simulink model "Lab1_parameter_estimation_student"  (R2025a)
settings: Solver=FixedStepAuto  StartTime=0.0  StopTime=20  FixedStep=0.0005  RelTol=1e-3
values from neighbouring files (symbols this model uses):
  motor_B = 3.13337426732843E-06    (= 3.13337426733e-06)    [Lab1_motor_params_student.m]    (also in Params_Chirp.mat = 6.5871616123e-07; Params_Ramp.mat = 8.73861222158e-05; Params_Sine.mat = 8.59415048861e-06; Params_Stair.mat = 3.2047e-05)
  motor_Eff = 0.750882138129295    (= 0.750882138129)    [Lab1_motor_params_student.m]    (also in Params_Chirp.mat = 0.998383269214; Params_Ramp.mat = 0.688800701516; Params_Sine.mat = 0.573625535666; Params_Stair.mat = 0.952868616)
  motor_J = 3.67584411965396E-06    (= 3.67584411965e-06)    [Lab1_motor_params_student.m]    (also in Params_Chirp.mat = 1.17123806047e-05; Params_Ramp.mat = 8.05298799031e-05; Params_Sine.mat = 8.20240322026e-06; Params_Stair.mat = 9.875e-06)
  motor_Ke = 0.0595281219387613    (= 0.0595281219388)    [Lab1_motor_params_student.m]    (also in Params_Chirp.mat = 0.0500817047826; Params_Ramp.mat = 0.0340798970374; Params_Sine.mat = 0.0488089871517; Params_Stair.mat = 0.047996267)
  motor_L = 0.136562826    [Lab1_motor_params_student.m]
  motor_R = 9.393179725    [Lab1_motor_params_student.m]
libraries: simulink x3
settings Model: Creator=tanawatp  LastModifiedBy=User
settings RTWCC: GPUComputeCapability=3.5

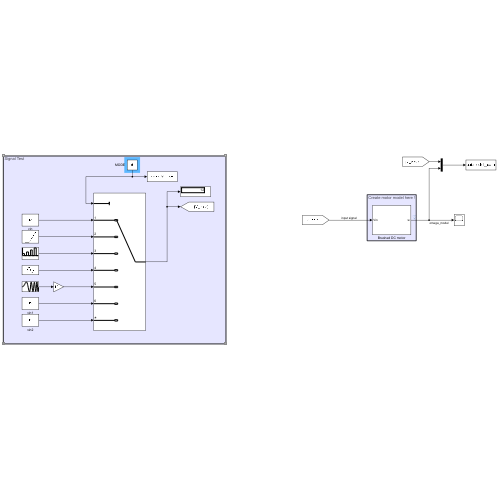
[thumbnail: Simulink's stored preview of the top-level diagram]
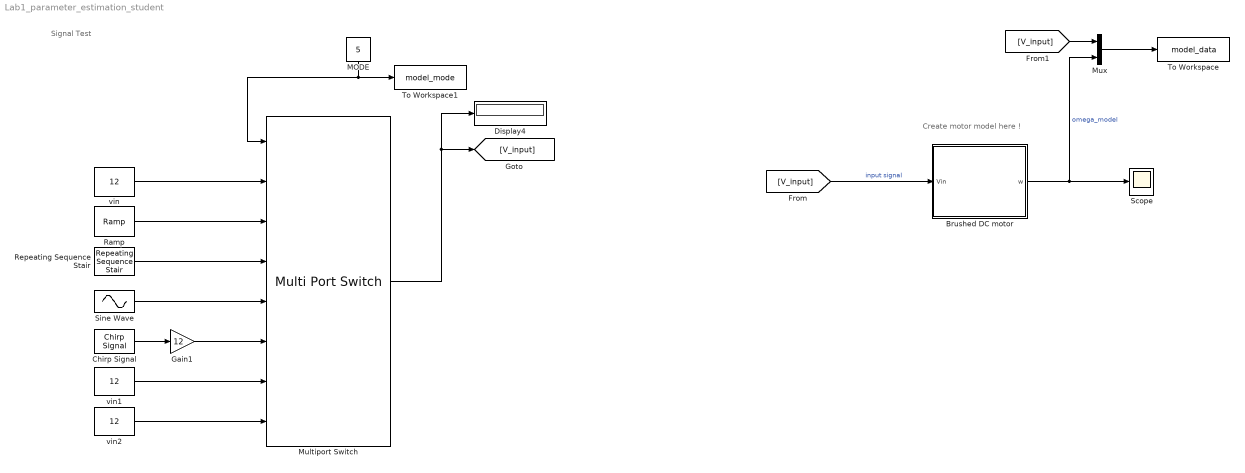
== system Lab1_parameter_estimation_student ==
  note: Create motor model here !
  note: Signal Test
  Brushed DC motor : Subsystem
  Chirp Signal : simulink/Sources/Chirp Signal  f1=0  T=20  f2=pi
  Display4 : Display
  Gain1 : Gain  Gain=12
  MODE : Constant  Value=5
  Multiport Switch : MultiPortSwitch  Inputs=6  DataPortForDefault=Additional data port  SaturateOnIntegerOverflow=off  InputSameDT=off
  Mux : Mux  Inputs=2
  Ramp : simulink/Sources/Ramp  slope=3  start=0  InitialOutput=0
  Repeating Sequence Stair : simulink/Sources/Repeating Sequence Stair  OutValues=[3 0 6 0 9 0 12 0]  tsamp=5  OutMin=[]  OutMax=[]  OutDataTypeStr=double  OutputDataTypeScalingMode=double  OutDataType=fixdt(0,8)  ConRadixGroup=Best Precision: Vector-wise  OutScaling=2^-12
  Scope : Scope
      settings: ActiveDisplayYMinimum=-26.38033  ActiveDisplayYMaximum=237.42293
  Sine Wave : Sin  Amplitude=12  Frequency=pi  SampleTime=0
  To Workspace : ToWorkspace  VariableName=model_data  SaveFormat=Timeseries  SampleTime=-1
  To Workspace1 : ToWorkspace  VariableName=model_mode  SaveFormat=Timeseries  SampleTime=-1
  vin : Constant  Value=12
  vin1 : Constant  Value=12
  vin2 : Constant  Value=12
  wires:
  Brushed DC motor/1(w) -> Mux/2, Scope/1  "omega_model"
  [V_input] -> Brushed DC motor/1(Vin)  "input signal"
  Multiport Switch/1 -> Display4/1, [V_input]
  [V_input] -> Mux/1
  Mux/1 -> To Workspace/1
  MODE/1 -> Multiport Switch/1, To Workspace1/1
  Sine Wave/1 -> Multiport Switch/5
  Ramp/1 -> Multiport Switch/3
  Repeating Sequence Stair/1 -> Multiport Switch/4
  Chirp Signal/1 -> Gain1/1
  vin/1 -> Multiport Switch/2
  Gain1/1 -> Multiport Switch/6
  vin1/1 -> Multiport Switch/7
  vin2/1 -> Multiport Switch/8

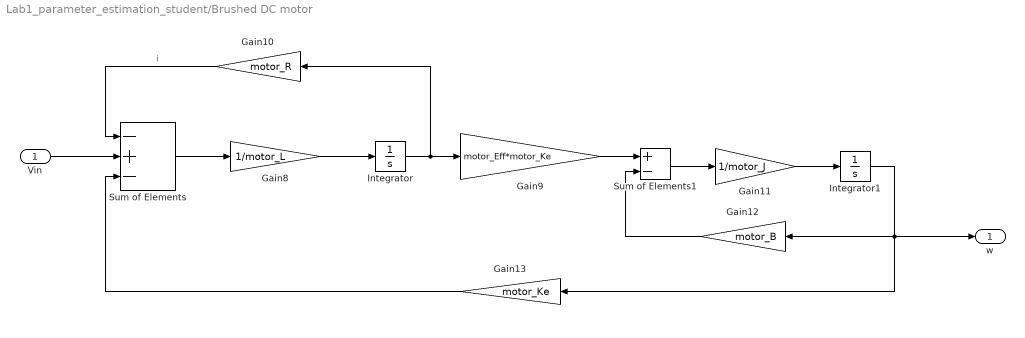
== system Lab1_parameter_estimation_student/Brushed DC motor ==
  Vin : Inport
  Gain10 : Gain  Gain=motor_R
  Gain11 : Gain  Gain=1/motor_J
  Gain12 : Gain  Gain=motor_B
  Gain13 : Gain  Gain=motor_Ke
  Gain8 : Gain  Gain=1/motor_L
  Gain9 : Gain  Gain=motor_Eff*motor_Ke
  Integrator : Integrator
  Integrator1 : Integrator
  Sum of Elements : Sum  Inputs=-+-
  Sum of Elements1 : Sum  Inputs=+-
  w : Outport
  wires:
  Sum of Elements/1 -> Gain8/1
  Gain8/1 -> Integrator/1
  Integrator/1 -> Gain9/1, Gain10/1
  Gain10/1 -> Sum of Elements/1  "i"
  Sum of Elements1/1 -> Gain11/1
  Gain9/1 -> Sum of Elements1/1
  Gain11/1 -> Integrator1/1
  Integrator1/1 -> w/1, Gain13/1, Gain12/1
  Gain12/1 -> Sum of Elements1/2
  Gain13/1 -> Sum of Elements/3
  Vin/1 -> Sum of Elements/2
